simulink model "psk"  (R2019a)
settings: Solver=VariableStepAuto  StartTime=0.0  StopTime=10.0  RelTol=1e-3
settings Model: Creator=dante  LastModifiedBy=dante

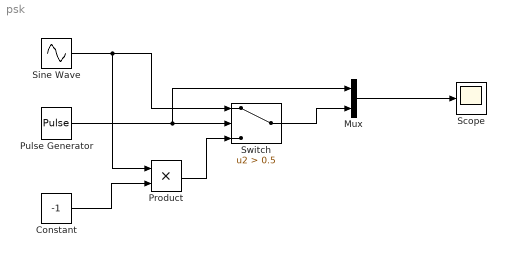
== system psk ==
  Constant : Constant  Value=-1
  Mux : Mux  Inputs=2
  Product : Product
  Pulse Generator : DiscretePulseGenerator  PulseType=Time based  PulseWidth=50
  Scope : Scope
  Sine Wave : Sin  Frequency=2*pi*2  SampleTime=0.01
  Switch : Switch  Criteria=u2 > Threshold  Threshold=0.5
  wires:
  Pulse Generator/1 -> Mux/1, Switch/2
  Sine Wave/1 -> Product/1, Switch/1
  Product/1 -> Switch/3
  Constant/1 -> Product/2
  Mux/1 -> Scope/1
  Switch/1 -> Mux/2
